simulink model "my_turn_stanley"  (R2020a)
settings: Solver=FixedStepAuto  StartTime=0.0  StopTime=6.7  FixedStep=0.05  RelTol=1e-3
libraries: simulink x1
settings Model: Creator=Jamie  LastModifiedBy=Jamie

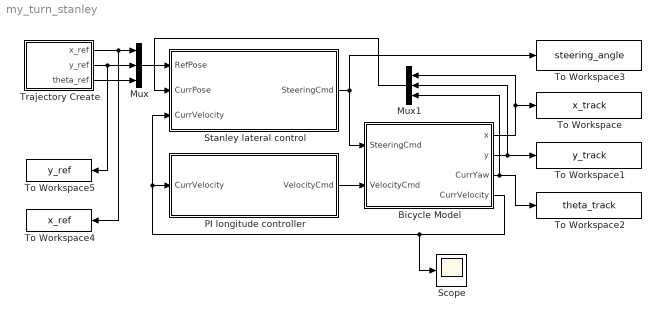
== system my_turn_stanley ==
  Bicycle Model : Subsystem
  Mux : Mux  Inputs=3
  Mux1 : Mux  Inputs=3
  PI longitude controller : Subsystem
  Scope : Scope
  Stanley lateral control : Subsystem
  To Workspace : ToWorkspace  VariableName=x_track  SampleTime=-1
      settings: Save2DSignal=2-D array (concatenate along first dimension)
  To Workspace1 : ToWorkspace  VariableName=y_track  SampleTime=-1
      settings: Save2DSignal=2-D array (concatenate along first dimension)
  To Workspace2 : ToWorkspace  VariableName=theta_track  SampleTime=-1
      settings: Save2DSignal=2-D array (concatenate along first dimension)
  To Workspace3 : ToWorkspace  VariableName=steering_angle  SampleTime=-1
      settings: Save2DSignal=2-D array (concatenate along first dimension)
  To Workspace4 : ToWorkspace  VariableName=x_ref  SampleTime=-1
      settings: Save2DSignal=2-D array (concatenate along first dimension)
  To Workspace5 : ToWorkspace  VariableName=y_ref  SampleTime=-1
      settings: Save2DSignal=2-D array (concatenate along first dimension)
  Trajectory Create : Subsystem
  wires:
  Stanley lateral control/1(SteeringCmd) -> Bicycle Model/1(SteeringCmd), To Workspace3/1
  Bicycle Model/3(CurrYaw) -> To Workspace2/1, Mux1/3
  Bicycle Model/1(x) -> Mux1/1, To Workspace/1
  Bicycle Model/2(y) -> To Workspace1/1, Mux1/2
  Bicycle Model/4(CurrVelocity) -> Scope/1, Stanley lateral control/3(CurrVelocity), PI longitude controller/1(CurrVelocity)
  Mux/1 -> Stanley lateral control/1(RefPose)
  Mux1/1 -> Stanley lateral control/2(CurrPose)
  PI longitude controller/1(VelocityCmd) -> Bicycle Model/2(VelocityCmd)
  Trajectory Create/1(x_ref) -> To Workspace4/1, Mux/1
  Trajectory Create/2(y_ref) -> To Workspace5/1, Mux/2
  Trajectory Create/3(theta_ref) -> Mux/3

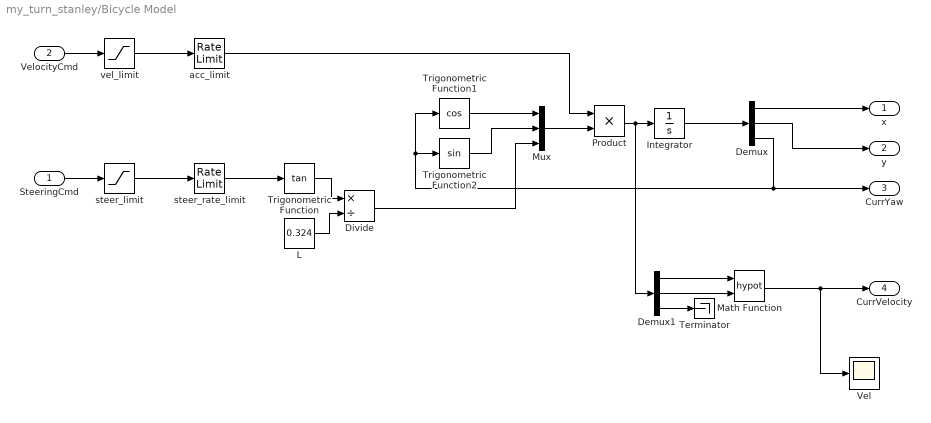
== system my_turn_stanley/Bicycle Model ==
  SteeringCmd : Inport
  VelocityCmd : Inport  Port=2
  Demux : Demux  Outputs=3
  Demux1 : Demux  Outputs=3
  Divide : Product  Inputs=*/
  Integrator : Integrator  InitialCondition=[0, 0, pi/2]
  L : Constant  Value=0.324
  Math Function : Math  Operator=hypot  SaturateOnIntegerOverflow=on
  Mux : Mux  Inputs=3
  Product : Product
  Terminator : Terminator
  Trigonometric Function : Trigonometry  Operator=tan
  Trigonometric Function1 : Trigonometry  Operator=cos
  Trigonometric Function2 : Trigonometry
  Vel : Scope
  acc_limit : RateLimiter  RisingSlewLimit=10  FallingSlewLimit=-10  SampleTimeMode=inherited
  steer_limit : Saturate
  steer_rate_limit : RateLimiter  RisingSlewLimit=20  FallingSlewLimit=-20  SampleTimeMode=inherited
  vel_limit : Saturate  UpperLimit=3  LowerLimit=-3
  x : Outport
  y : Outport  Port=2
  CurrYaw : Outport  Port=3
  CurrVelocity : Outport  Port=4
  wires:
  SteeringCmd/1 -> steer_limit/1
  VelocityCmd/1 -> vel_limit/1
  vel_limit/1 -> acc_limit/1
  steer_limit/1 -> steer_rate_limit/1
  steer_rate_limit/1 -> Trigonometric Function/1
  Trigonometric Function/1 -> Divide/1
  L/1 -> Divide/2
  acc_limit/1 -> Product/1
  Trigonometric Function1/1 -> Mux/1
  Trigonometric Function2/1 -> Mux/2
  Mux/1 -> Product/2
  Product/1 -> Demux1/1, Integrator/1
  Divide/1 -> Mux/3
  Integrator/1 -> Demux/1
  Demux/1 -> x/1
  Demux/2 -> y/1
  Demux/3 -> Trigonometric Function1/1, Trigonometric Function2/1, CurrYaw/1
  Demux1/1 -> Math Function/1
  Demux1/2 -> Math Function/2
  Demux1/3 -> Terminator/1
  Math Function/1 -> Vel/1, CurrVelocity/1

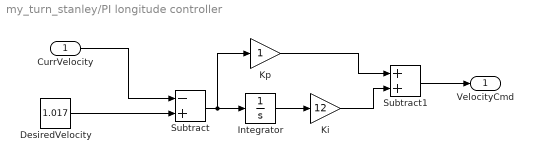
== system my_turn_stanley/PI longitude controller ==
  CurrVelocity : Inport
  DesiredVelocity : Constant  Value=1.017
  Integrator : Integrator
  Ki : Gain  Gain=12
  Kp : Gain
  Subtract : Sum  Inputs=-+
  Subtract1 : Sum
  VelocityCmd : Outport
  wires:
  Subtract1/1 -> VelocityCmd/1
  DesiredVelocity/1 -> Subtract/2
  Ki/1 -> Subtract1/2
  Subtract/1 -> Integrator/1, Kp/1
  Integrator/1 -> Ki/1
  Kp/1 -> Subtract1/1
  CurrVelocity/1 -> Subtract/1

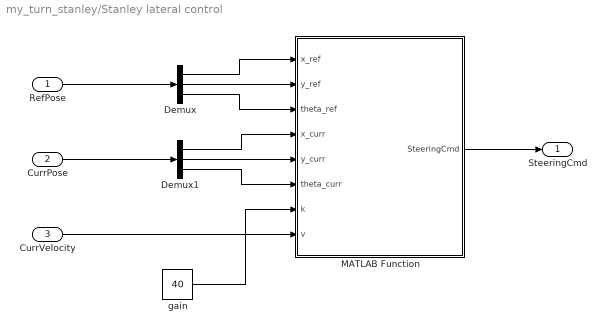
== system my_turn_stanley/Stanley lateral control ==
  RefPose : Inport
  CurrPose : Inport  Port=2
  CurrVelocity : Inport  Port=3
  Demux : Demux  Outputs=3
  Demux1 : Demux  Outputs=3
  MATLAB Function : MATLAB Function  TreatAsAtomicUnit=on
  gain : Constant  Value=40
  SteeringCmd : Outport
  wires:
  RefPose/1 -> Demux/1
  MATLAB Function/1(SteeringCmd) -> SteeringCmd/1
  Demux/1 -> MATLAB Function/1(x_ref)
  Demux/2 -> MATLAB Function/2(y_ref)
  Demux/3 -> MATLAB Function/3(theta_ref)
  Demux1/1 -> MATLAB Function/4(x_curr)
  Demux1/2 -> MATLAB Function/5(y_curr)
  Demux1/3 -> MATLAB Function/6(theta_curr)
  CurrPose/1 -> Demux1/1
  CurrVelocity/1 -> MATLAB Function/8(v)
  gain/1 -> MATLAB Function/7(k)

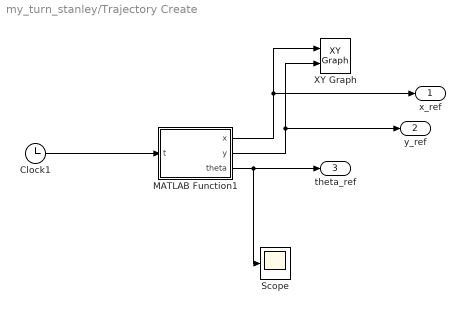
== system my_turn_stanley/Trajectory Create ==
  Clock1 : Clock
  MATLAB Function1 : MATLAB Function  TreatAsAtomicUnit=on
  Scope : Scope
  XY Graph : simulink/Sinks/XY Graph  xmin=-1  xmax=1  ymin=-1  ymax=1  st=-1
  x_ref : Outport
  y_ref : Outport  Port=2
  theta_ref : Outport  Port=3
  wires:
  MATLAB Function1/1(x) -> XY Graph/1, x_ref/1
  MATLAB Function1/3(theta) -> Scope/1, theta_ref/1
  MATLAB Function1/2(y) -> XY Graph/2, y_ref/1
  Clock1/1 -> MATLAB Function1/1(t)

== matlab function my_turn_stanley/Stanley lateral control/MATLAB Function ==
  data: x_ref input; SteeringCmd output; y_ref input; theta_ref input; x_curr input; y_curr input; theta_curr input; k input; v input
function SteeringCmd = fcn(x_ref, y_ref, theta_ref, x_curr, y_curr, theta_curr, k, v)

e_crosstrack = x_curr*sin(theta_ref) - y_curr*cos(theta_ref) - x_ref*sin(theta_ref) + y_ref*cos(theta_ref);

e_heading = theta_ref - theta_curr;

SteeringCmd = e_heading + atan(k*e_crosstrack/(0.1 + v));

== matlab function my_turn_stanley/Trajectory Create/MATLAB Function1 ==
  data: x output; t input; y output; theta output
function [x, y, theta] = fcn(t)

R = 1.5;
v = 1;

if ((t >= 0)&&(t <= 1))
    x = 0;
    y = t;
    theta = pi/2;
elseif((t >= 1)&&(t <= 1+R*pi/v))
    x = 1.5 - 1.5*cos(v/R*(t-1));
    y = 1 + 1.5*sin(v/R*(t-1));
    theta = pi/2 - 2*(t - 1)/3;
elseif ((t >= 1 + R*pi/v)&&(t <= 2+R*pi/v))
    x = 3;
    y = -t + 2+1.5*pi/v;
    theta = -pi/2;
else
    x = 3;
    y = 0;
    theta = -pi/2;
end
end
